simulink model "VariousSpeed2018_14dof_ypredictor_sc"  (R2017a)
settings: Solver=ode4  StartTime=0.0  StopTime=70  FixedStep=dt  RelTol=1e-3
values from neighbouring files (symbols this model uses):
  g_motor_eff = 1    [VESIM_init.m]
  gr_motor = 0    [VESIM_init.m]
undefined symbols (not defined in the file or in its folder): A_mc, brake_Pw, brake_V, C_q, diff_efficiency, diff_wRatio, dt, engine_inertia, error_lookuptable, F_cf, F_cs, fmin_mg, fmin_mg_na, J_cal, K_vb, Kp_rpm, mdot_fuel, model_lookuptable, no_cyl, P_0, P_gain, rpm0_c, rpm2rads, rpm_e, rpm_hi_idle, rpm_idle, rpm_max_c, rpm_rated, Standard_Devices, Ti_rpm, torque_engine, trq_scale, Tt_rpm, UDP_Protocol, vdes, Xobs, Yobs
libraries: simulink x10, vrlib x3, sldrtlib x3, SimulinkExecutionControl x1
(part 2 of 2)

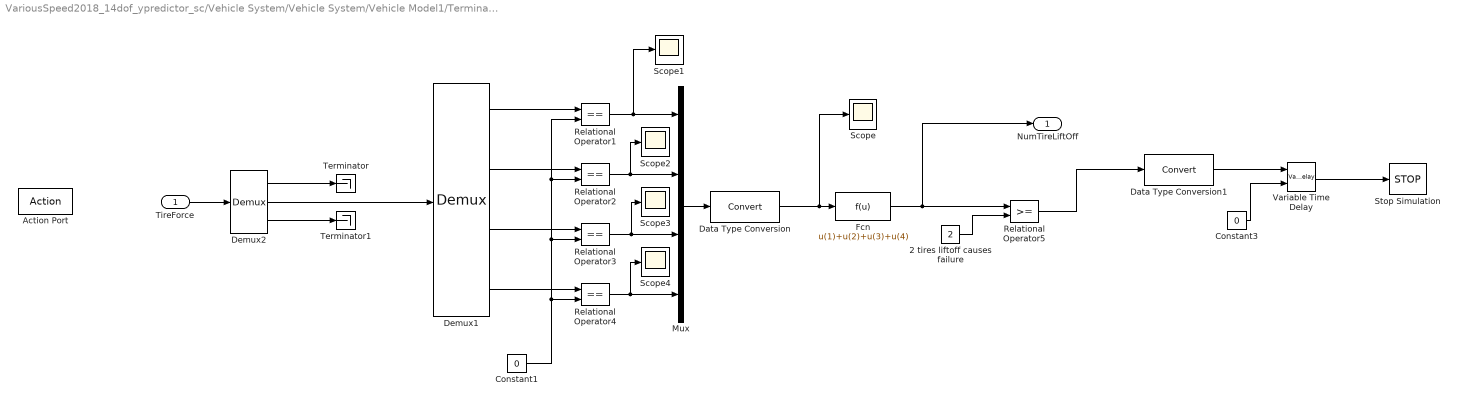
== system VariousSpeed2018_14dof_ypredictor_sc/Vehicle System/Vehicle System/Vehicle Model1/Terminate if vehicle tire lift-off ==
  TireForce : Inport
  Action Port : ActionPort
  2 tires liftoff causes failure : Constant  Value=2
  Constant1 : Constant  Value=0
  Constant3 : Constant  Value=0
  Data Type Conversion : DataTypeConversion
  Data Type Conversion1 : DataTypeConversion
  Demux1 : Demux
  Demux2 : Demux  Outputs=[8,4,17]
  Fcn : Fcn  Expr=u(1)+u(2)+u(3)+u(4)
  Mux : Mux
  Relational Operator{1..4} (4 alike) : RelationalOperator  Operator===  RndMeth=Nearest  InputSameDT=on
  Relational Operator5 : RelationalOperator  RndMeth=Nearest  InputSameDT=on
  Scope{,1..4} (5 alike) : Scope
  Stop Simulation : Stop
  Terminator : Terminator
  Terminator1 : Terminator
  Variable Time Delay : VariableTransportDelay  MaximumDelay=10  MaximumPoints=10000
  NumTireLiftOff : Outport  InitialOutput=0
  wires:
  Demux2/1 -> Terminator/1
  Demux2/3 -> Terminator1/1
  Demux2/2 -> Demux1/1
  TireForce/1 -> Demux2/1
  Demux1/1 -> Relational Operator1/1
  Demux1/2 -> Relational Operator2/1
  Demux1/3 -> Relational Operator3/1
  Demux1/4 -> Relational Operator4/1
  Relational Operator1/1 -> Scope1/1, Mux/1
  Relational Operator2/1 -> Scope2/1, Mux/2
  Relational Operator3/1 -> Scope3/1, Mux/3
  Relational Operator4/1 -> Scope4/1, Mux/4
  2 tires liftoff causes failure/1 -> Relational Operator5/2
  Mux/1 -> Data Type Conversion/1
  Data Type Conversion/1 -> Scope/1, Fcn/1
  Relational Operator5/1 -> Data Type Conversion1/1
  Constant1/1 -> Relational Operator2/2, Relational Operator1/2, Relational Operator3/2, Relational Operator4/2
  Fcn/1 -> NumTireLiftOff/1, Relational Operator5/1
  Variable Time Delay/1 -> Stop Simulation/1
  Constant3/1 -> Variable Time Delay/2
  Data Type Conversion1/1 -> Variable Time Delay/1

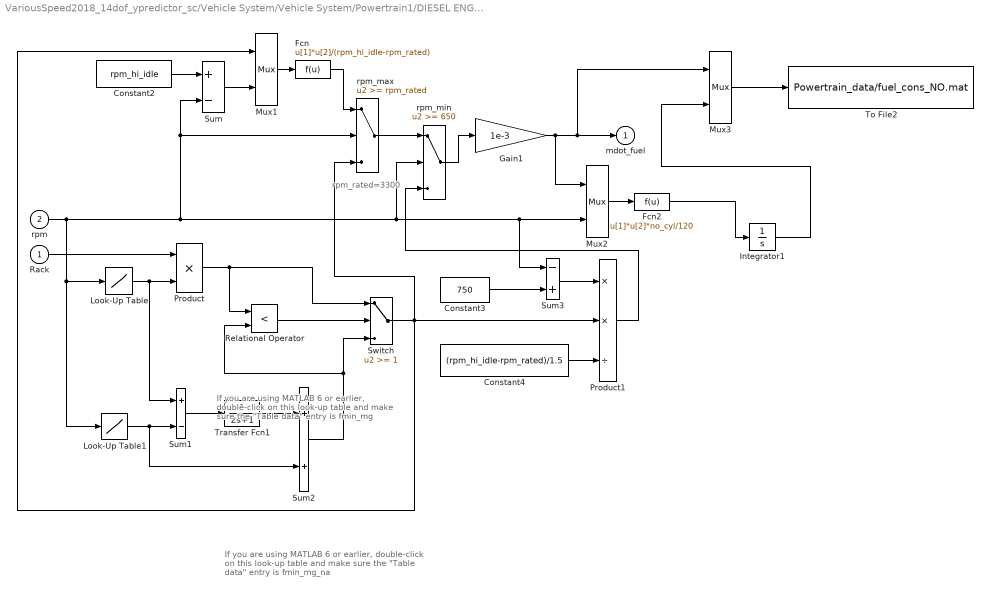
== system VariousSpeed2018_14dof_ypredictor_sc/Vehicle System/Vehicle System/Powertrain1/DIESEL ENGINE/Fuel controller// Governor ==
  note: If you are using MATLAB 6 or earlier,
      | double-click on this look-up table and
      | make sure the "Table data" entry is fmin_mg
  note: If you are using MATLAB 6 or earlier,
      | double-click on this look-up table and
      | make sure the "Table data" entry is fmin_mg_na
  note: rpm_rated=3300
  Rack : Inport
  rpm : Inport  Port=2
  Constant2 : Constant  Value=rpm_hi_idle
  Constant3 : Constant  Value=750
  Constant4 : Constant  Value=(rpm_hi_idle-rpm_rated)/1.5
  Fcn : Fcn  Expr=u[1]*u[2]/(rpm_hi_idle-rpm_rated)
  Fcn2 : Fcn  Expr=u[1]*u[2]*no_cyl/120
  Gain1 : Gain  Gain=1e-3  SaturateOnIntegerOverflow=on  OutDataTypeStr=Inherit: Same as input  ParamDataTypeStr=Inherit: Same as input
  Integrator1 : Integrator
  Look-Up Table : Lookup  InputValues=rpm_e  Table=fmin_mg  SaturateOnIntegerOverflow=on
  Look-Up Table1 : Lookup  InputValues=rpm_e  Table=fmin_mg_na  SaturateOnIntegerOverflow=on
  Mux1 : Mux  Inputs=2
  Mux2 : Mux  Inputs=2
  Mux3 : Mux  Inputs=2
  Product : Product  SaturateOnIntegerOverflow=on  InputSameDT=on  OutDataTypeStr=Inherit: Same as first input
  Product1 : Product  Inputs=**/  SaturateOnIntegerOverflow=on  InputSameDT=on  OutDataTypeStr=Inherit: Same as first input
  Relational Operator : RelationalOperator  Operator=<  RndMeth=Nearest  InputSameDT=on
  Sum : Sum  Inputs=+-  SaturateOnIntegerOverflow=on  InputSameDT=on  OutDataTypeStr=Inherit: Same as first input
  Sum1 : Sum  Inputs=+-  SaturateOnIntegerOverflow=on  InputSameDT=on  OutDataTypeStr=Inherit: Same as first input
  Sum2 : Sum  SaturateOnIntegerOverflow=on  InputSameDT=on  OutDataTypeStr=Inherit: Same as first input
  Sum3 : Sum  Inputs=-+  SaturateOnIntegerOverflow=on  InputSameDT=on  OutDataTypeStr=Inherit: Same as first input
  Switch : Switch  Threshold=1  SaturateOnIntegerOverflow=on  InputSameDT=on
  To File2 : ToFile  Filename=Powertrain_data/fuel_cons_NO.mat  MatrixName=fuel_cons
  Transfer Fcn1 : TransferFcn  Denominator=[2 1]
  rpm_max : Switch  Threshold=rpm_rated  SaturateOnIntegerOverflow=on  InputSameDT=on
  rpm_min : Switch  Threshold=650  SaturateOnIntegerOverflow=on  InputSameDT=on
  mdot_fuel : Outport  InitialOutput=0
  wires:
  Mux3/1 -> To File2/1
  Integrator1/1 -> Mux3/2
  Fcn2/1 -> Integrator1/1
  Switch/1 -> rpm_max/3, Product1/2, Mux1/1
  Product/1 -> Switch/1, Relational Operator/1
  Sum2/1 -> Relational Operator/2, Switch/3
  Relational Operator/1 -> Switch/2
  Look-Up Table1/1 -> Sum2/2, Sum1/2
  Transfer Fcn1/1 -> Sum2/1
  Look-Up Table/1 -> Product/2, Sum1/1
  Sum1/1 -> Transfer Fcn1/1
  Rack/1 -> Product/1
  rpm/1 -> rpm_max/2, Sum/2, Sum3/1, Mux2/2, rpm_min/2, Look-Up Table/1, Look-Up Table1/1
  Fcn/1 -> rpm_max/1
  rpm_max/1 -> rpm_min/1
  Product1/1 -> rpm_min/3
  Constant4/1 -> Product1/3
  Sum3/1 -> Product1/1
  Constant3/1 -> Sum3/2
  Constant2/1 -> Sum/1
  rpm_min/1 -> Gain1/1
  Mux2/1 -> Fcn2/1
  Gain1/1 -> Mux3/1, mdot_fuel/1, Mux2/1
  Sum/1 -> Mux1/2
  Mux1/1 -> Fcn/1

== system VariousSpeed2018_14dof_ypredictor_sc/Vehicle System/Vehicle System/Powertrain1/DIESEL ENGINE/Idle Controller ==
  note: 1/0.6464
  note: 2.7013
  note: 1/(3300-1000)
  note: 750 RPM
  note: anti-windup gain
  note: integral gain
  note: proportional gain
  engine speed : Inport
  driver command : Inport  Port=2
  Gain6 : Gain  Gain=Kp_rpm  SaturateOnIntegerOverflow=on  OutDataTypeStr=Inherit: Same as input  ParamDataTypeStr=Inherit: Same as input
  Gain7 : Gain  Gain=1/Ti_rpm  SaturateOnIntegerOverflow=on  OutDataTypeStr=Inherit: Same as input  ParamDataTypeStr=Inherit: Same as input
  Gain8 : Gain  Gain=1/(rpm_max_c-rpm0_c)  SaturateOnIntegerOverflow=on  OutDataTypeStr=Inherit: Same as input  ParamDataTypeStr=Inherit: Same as input
  Gain9 : Gain  Gain=1/Tt_rpm  SaturateOnIntegerOverflow=on  OutDataTypeStr=Inherit: Same as input  ParamDataTypeStr=Inherit: Same as input
  Idle speed : Constant  Value=rpm_idle
  Integrator2 : Integrator
  Saturation2 : Saturate  UpperLimit=1  LowerLimit=0.005
  Sum5 : Sum  Inputs=-+  SaturateOnIntegerOverflow=on  InputSameDT=on  OutDataTypeStr=Inherit: Same as first input
  Sum6 : Sum  SaturateOnIntegerOverflow=on  InputSameDT=on  OutDataTypeStr=Inherit: Same as first input
  Sum7 : Sum  Inputs=+-  SaturateOnIntegerOverflow=on  InputSameDT=on  OutDataTypeStr=Inherit: Same as first input
  Sum8 : Sum  SaturateOnIntegerOverflow=on  InputSameDT=on  OutDataTypeStr=Inherit: Same as first input
  Switch : Switch  Threshold=.11  SaturateOnIntegerOverflow=on  InputSameDT=on
  rack : Outport
  wires:
  Gain8/1 -> Gain6/1
  Sum7/1 -> Gain8/1
  engine speed/1 -> Sum7/2
  Idle speed/1 -> Sum7/1
  Saturation2/1 -> Sum5/2, rack/1
  driver command/1 -> Switch/2, Switch/1
  Switch/1 -> Sum5/1, Saturation2/1
  Sum6/1 -> Switch/3
  Gain9/1 -> Sum8/2
  Integrator2/1 -> Sum6/2
  Sum8/1 -> Integrator2/1
  Gain7/1 -> Sum8/1
  Sum5/1 -> Gain9/1
  Gain6/1 -> Gain7/1, Sum6/1

== system VariousSpeed2018_14dof_ypredictor_sc/Vehicle System/Vehicle System/Powertrain1/DRIVELINE/Drivetrain1 ==
  demand : Inport
  pump_f : Inport  Port=2
  shaft_f : Inport  Port=3
  Demux : Demux  Outputs=[1 1 1 1 1 1 1 1 1 1 1 1 1 ]
  Mux : Mux  Inputs=[1 1 1 ]
  S-Function : S-Function  FunctionName=Drivetrain  SFunctionDeploymentMode=off  EnableBusSupport=off
  gear_out : Outport
  gear_ratio_w : Outport  Port=2
  pump_e : Outport  Port=3
  shaft_e : Outport  Port=4
  stateDerTransC : Outport  Port=5
  stateDerTransI : Outport  Port=6
  stateTransC : Outport  Port=7
  stateTransI : Outport  Port=8
  trans_T_ratio_out : Outport  Port=9
  T_turbine_out : Outport  Port=10
  w_out_trans_out : Outport  Port=11
  w_ratio_disp : Outport  Port=12
  w_Turbine_out : Outport  Port=13
  wires:
  demand/1 -> Mux/1
  pump_f/1 -> Mux/2
  shaft_f/1 -> Mux/3
  Demux/1 -> gear_out/1
  Demux/2 -> gear_ratio_w/1
  Demux/3 -> pump_e/1
  Demux/4 -> shaft_e/1
  Demux/5 -> stateDerTransC/1
  Demux/6 -> stateDerTransI/1
  Demux/7 -> stateTransC/1
  Demux/8 -> stateTransI/1
  Demux/9 -> trans_T_ratio_out/1
  Demux/10 -> T_turbine_out/1
  Demux/11 -> w_out_trans_out/1
  Demux/12 -> w_ratio_disp/1
  Demux/13 -> w_Turbine_out/1
  Mux/1 -> S-Function/1
  S-Function/1 -> Demux/1

== system VariousSpeed2018_14dof_ypredictor_sc/Vehicle System/Vehicle System/Powertrain1/DRIVELINE/engine dynamics (flywheel inertia only) ==
  brake torque : Inport
  Load Torque : Inport  Port=2
  Engine polar moment of inertia1 : Constant  Value=engine_inertia
  Mux : Mux  Inputs=2
  Sum : Sum  Inputs=+-  SaturateOnIntegerOverflow=on  InputSameDT=on  OutDataTypeStr=Inherit: Same as first input
  calculate omega (replace current init val with value from input file) : Integrator  InitialCondition=0.01*2*pi/60
  div : Fcn  Expr=u[1]/u[2]
  rad/s : Outport  InitialOutput=0
  wires:
  Mux/1 -> div/1
  Sum/1 -> Mux/1
  Load Torque/1 -> Sum/2
  Engine polar moment of inertia1/1 -> Mux/2
  brake torque/1 -> Sum/1
  calculate omega (replace current init val with value from input file)/1 -> rad/s/1
  div/1 -> calculate omega (replace current init val with value from input file)/1

== matlab function VariousSpeed2018_14dof_ypredictor_sc/Autonomy/MATLAB Function4 ==
  data: u input; y output
function y = fcn(u)

y = u(u(104));

== matlab function VariousSpeed2018_14dof_ypredictor_sc/Autonomy/MATLAB Function ==
  data: u input; y output
function y = fcn(u)

y = u(min(u(104)+25,101));

== matlab function VariousSpeed2018_14dof_ypredictor_sc/Vehicle System/MATLAB Function ==
  data: u input; y output
function y = fcn(u)

y = 170*sin(0.005*u)+280*sin(0.001*u)+50*cos(0.02*u)-50;

== matlab function VariousSpeed2018_14dof_ypredictor_sc/Autonomy/MATLAB Function1 ==
  data: u input; y output
function y = fcn(u)
N = 51;
y = u(N+1);

== matlab function VariousSpeed2018_14dof_ypredictor_sc/Autonomy/MATLAB Function2 ==
  data: u input; y output
function y = fcn(u)

N = 51;
y = u(N+4);

== matlab function VariousSpeed2018_14dof_ypredictor_sc/Haptic Shared Control/Trigger1/MATLAB Function ==
  data: u input; vect output size=[1 10]; vect_old input; tr_vect_old input; threshold input; flag output; tr_vect output size=[1 20]; trigger output
function [vect, flag, tr_vect, trigger] = fcn(u, vect_old, tr_vect_old, threshold)
    vect = zeros(1,10); 
    vect(1,1) = u;
    vect(1,2:10) = vect_old(1:9);
    vect_ordered = sort(vect);
    
    if mean(vect_ordered(1:2)) > threshold
        flag = 1;
    else
        flag = 0;
    end
    
    tr_vect = zeros(1,20);
    tr_vect(1,1) = flag;
    tr_vect(1, 2:20) = tr_vect_old(1:19);
    if sum(tr_vect) == 20
        trigger = 1;
    else
        trigger = 0;
    end
end

== matlab function VariousSpeed2018_14dof_ypredictor_sc/Autonomy/Subsystem/Distance Indicator/Subsystem1/MATLAB Function ==
  data: Xv input; Xinit_final output; Yv input; Xinit input; alpha input; distance output
function [Xinit_final, distance] = DistanceIndicator(Xv, Yv, Xinit, alpha)

    threshold = 0.0005;
    Yinit = 170*sin(0.005*Xinit) + 280*sin(0.001*Xinit) + 50*cos(0.02*Xinit) - 50;
    Yd = 170*0.005*cos(0.005*Xinit) + 280*0.001*cos(0.001*Xinit) - 50*0.02*sin(0.02*Xinit);
    Ydd = -170*0.005*0.005*sin(0.005*Xinit) - 280*0.001*0.001*sin(0.001*Xinit) - 50*0.02*0.02*cos(0.02*Xinit);
    
    Proj = ((Xv - Xinit) + Yd * (Yv - Yinit))/sqrt(1 + Yd^2);
    Projd = (((-1 + Ydd * (Yv - Yinit) - (Yd)^2) * sqrt(1 + Yd^2)) - ((Xv - Xinit + Yd*(Yv - Yinit))) * 1/2 * (1+Yd^2)^(-1/2) * 2 * Yd * Ydd)/(1 + Yd^2);
    
    iter = 1;
    Move = 2 * Proj * Projd;
    
    while (abs(Move * alpha) >= threshold) && (iter <= 1000)
        Xinit = Xinit - alpha * Move;
        Yinit = 170*sin(0.005*Xinit) + 280*sin(0.001*Xinit) + 50*cos(0.02*Xinit) - 50;
        Yd = 170*0.005*cos(0.005*Xinit) + 280*0.001*cos(0.001*Xinit) - 50*0.02*sin(0.02*Xinit);
        Ydd = -170*0.005*0.005*sin(0.005*Xinit) - 280*0.001*0.001*sin(0.001*Xinit) - 50*0.02*0.02*cos(0.02*Xinit);
    
        Proj = ((Xv - Xinit) + Yd * (Yv - Yinit))/sqrt(1 + Yd^2);
        Projd = (((-1 + Ydd * (Yv - Yinit) - (Yd)^2) * sqrt(1 + Yd^2)) - ((Xv - Xinit + Yd*(Yv - Yinit))) * 1/2 * (1+Yd^2)^(-1/2) * 2 * Yd * Ydd)/(1 + Yd^2);
        Move = 2 * Proj * Projd;
        iter = iter + 1;
    end
    
    Xinit_final = Xinit;
    distance = sqrt((Xinit - Xv)^2 + (Yinit - Yv)^2);
end

== matlab function VariousSpeed2018_14dof_ypredictor_sc/Haptic Shared Control/Force Generator/Reference Governor/MATLAB Function ==
  data: ST_C input; ST_RG output; ST_L input
function ST_RG = fcn(ST_C, ST_L)
% ST_d = abs(ST_C - ST_L);
% if ST_d < 0.00075
%     ST_RG = ST_C;
% elseif ST_d < 0.00125
%     ST_RG = ST_L + 0.75*(ST_C - ST_L);
% elseif ST_d < 0.0016
%     ST_RG = ST_L + 0.5*(ST_C - ST_L);
% else
%     ST_RG = ST_L + 0.0016*(ST_C - ST_L)/ST_d;
ST_d = abs(ST_C - ST_L);
ST_diff = ST_C - ST_L;
    if ST_d < 0.0012
        ST_RG = ST_C;
    else
        add_diff = min(ST_d * 0.5, 0.0012) * ST_diff / ST_d;
        ST_RG = ST_L + add_diff;
    end

end

== matlab function VariousSpeed2018_14dof_ypredictor_sc/Vehicle System/Subsystem/MATLAB Function2 ==
  data: X0 input; ST_length input; X0predicted output; SP_length input; time_step input; idx input; dt input; st_old input; sp_old input
function X0predicted = fcn(X0, ST_length, SP_length, time_step, idx, dt, st_old, sp_old)
x0 = X0(1);
y0 = X0(2);
vy0 = X0(3);
dpsi = X0(4);
psi = X0(5);
if time_step == 0
    X0predicted = X0;
else
    if idx >= 1 
        st = ST_length(idx);
        vdes = SP_length(idx);
    else
        st = st_old;
        vdes = sp_old;
    end
    for i = 1:time_step
        four_dot = dotcalculator(st,vdes,x0,y0,vy0,dpsi,psi);
        if idx + i > 101
            st = ST_length(101);
            vdes = SP_length(101);
        else
            st = ST_length(idx+i);
            vdes = SP_length(idx+i);
        end
        x0 = x0 + dt * four_dot(1);
        y0 = y0 + dt * four_dot(2);
        vy0 = vy0 + dt * four_dot(3);
        dpsi = dpsi + dt * four_dot(4);
        psi = psi + dt * dpsi;
    end
    if idx + time_step > 101
        X0predicted = [x0; y0; vy0; dpsi; psi; ST_length(101); SP_length(101); 0];
    else
        a = idx+time_step;
        if a > 1
            X0predicted = [x0; y0; vy0; dpsi; psi; ST_length(a); SP_length(a); (SP_length(a) - SP_length(a-1))/dt];
        elseif a == 1
            X0predicted = [x0; y0; vy0; dpsi; psi; ST_length(a); SP_length(a); (SP_length(a) - sp_old)/dt];
        else
            X0predicted = [x0; y0; vy0; dpsi; psi; st_old; sp_old; (sp_old - vdes)/dt];
        end
    end
end
  


function fourdot = dotcalculator(st,vdes,x0,y0,vy0,dpsi,psi)
    % define model parameters
    m          = 2.6887e+03;
    Izz        = 4.1101e+03;
    la         = 1.5775;      % distance from CoG to front axle
    lb         = 1.7245;        % distance from CoG to rear axle
    FzF0       = 1.3680e+04;
    FzR0       = 1.2696e+04;
    dFzx_coeff = 705.;
    KZX        = 705.;
    KZYR       = 1040.;

    % defines polynominal for acceleration bounds
    AXC= [-0.000128015180401862,	0.00858618595422724,	-0.225657108071454,	3.08283259993589,	-0.000138537090018958,	0.00684702729623608,	-0.120391102052425,	-3.55886697370079];

    % vehicle Limits
    x_min    = 0.;
    x_max    = 400.;
    y_min    = 0.;
    y_max    = 400.;
    sa_min   = -30*pi/180;
    sa_max   = 30*pi/180;
    psi_min  = -2*pi;
    psi_max  = 2*pi;
    u_min    = 5.;   %5.
    u_max    = 29.;
    sr_min   = -5*pi/180;
    sr_max   = 5*pi/180;
    jx_min   = -5.;
    jx_max   = 5.;

    % tire parameters
    FZ0     = 35000.0;
    PCY1    = 1.5874;               %Shape factor Cfy for lateral forces
    PDY1    = 0.73957;              %Lateral friction Muy
    PDY2    = -0.075004;            %Variation of friction Muy with load
    PEY1    = 0.37562;              %Lateral curvature Efy at Fznom
    PEY2    = -0.069325;            %Variation of curvature Efy with load
    PEY3    = 0.29168;              %Zero order camber dependency of curvature Efy
    PKY1    = -10.289;              %Maximum value of stiffness Kfy/Fznom
    PKY2    = 3.3343;               %Load at which Kfy reaches maximum value
    PHY1    = 0.0056509;            %Horizontal shift Shy at Fznom
    PHY2    = -0.0020257;           %Variation of shift Shy with load
    PVY1    = 0.015216;             %Vertical shift in Svy/Fz at Fznom
    PVY2    = -0.010365;            %Variation of shift Svy/Fz with load
    PC1     = PCY1;
    PD1     = PDY1 - PDY2;
    PD2     = PDY2/FZ0;
    PE1     = PEY1 - PEY2;
    PE2     = PEY2/FZ0;
    PE3     = PEY3;
    PK1     = PKY1*FZ0;
    PK2     = 1/(PKY2*FZ0);
    PH1     = PHY1 - PHY2;
    PH2     = PHY2/FZ0;
    PV1     = PVY1 - PVY2;
    PV2     = PVY2/FZ0;

    Caf =  -8.4138e+04;	% cornering stiffness--front axle (N/rad)
    Car =  -7.8126e+04;	% cornering stiffness-- rear axle (N/rad)
    Fyf_min = -7500;
    Fyf_max = 7500;
    % constrained initial states
    x0_     = 0.;
    y0_     = 0.;
    psi0_   = 0.8464;
    v0_     = 0.;
    u0_     = 10.;
    sa0_    = 0.;
    sr0_    = 0.;
    ax0_    = 0.;
    jx0_    = 0.;
    r0_     = 0.;

    %%TODO: Move some of these parameters somewhere else
    % weights
    w_goal = 1.; % should be zero when vehicle is not within goal distance during prediction horizon
    w_psi  = 0.01;
    w_time = 0.05;
    w_haf  = 1.0e-5;
    w_Fz   = 0.1;  %0.5 in paper
    w_ce   = 1.;
    w_sa   = 0.1;
    w_sr   = 1.;
    w_jx   = 0.01;

    sm      = 5.; % (m) distance to make sure we don't hit obstacle
    Fz_min  = 1000.;
    Fz_off  = 100.;
    a_t     = Fz_min + 3*Fz_off;  % soft tire force constraint constants
    b_t     = Fz_off;
    EP      = 0.001;

    % other parameters
    L_Rd      = 5.;       % relaxation constant for LiDAR range (m)
    L_R       = 100.;     % LiDAR range (m)
    sigma     = 1.;       % 0.05 (m)small margin, if the vehicle is within this margin, then the target is considered to be reached

    
r=dpsi;    
v=vy0;    
ax=0;
ux=vdes;
sa=st;
FYF=( (PD2*(FzF0 - (ax - v*r)*dFzx_coeff)^2 + PD1*(FzF0 - (ax - v*r)*dFzx_coeff))*sin(PC1*atan((((PK1*sin(2*atan(PK2*(FzF0 - (ax - v*r)*dFzx_coeff))))/(((PD2*PC1*(FzF0 - (ax - v*r)*dFzx_coeff)^2 + PD1*PC1*(FzF0 - (ax - v*r)*dFzx_coeff)) + ((PD2*PC1*(FzF0 - (ax - v*r)*dFzx_coeff)^2 + PD1*PC1*(FzF0 - (ax - v*r)*dFzx_coeff)))/(((PD2*PC1*(FzF0 - (ax - v*r)*dFzx_coeff)^2 + PD1*PC1*(FzF0 - (ax - v*r)*dFzx_coeff))^2 + EP^2)^(0.5))*0.001)+EP))*((atan((v + la*r)/(ux+EP)) - sa) + PH2*(FzF0 - (ax - v*r)*dFzx_coeff) + PH1)) - ((PE2*(FzF0 - (ax - v*r)*dFzx_coeff) + PE1)*(1 - PE3)*(((atan((v + la*r)/(ux+EP)) - sa) + PH2*(FzF0 - (ax - v*r)*dFzx_coeff) + PH1))/((((atan((v + la*r)/(ux+EP)) - sa) + PH2*(FzF0 - (ax - v*r)*dFzx_coeff) + PH1)^2 + EP^2)^(0.5)))*((((PK1*sin(2*atan(PK2*(FzF0 - (ax - v*r)*dFzx_coeff))))/(((PD2*PC1*(FzF0 - (ax - v*r)*dFzx_coeff)^2 + PD1*PC1*(FzF0 - (ax - v*r)*dFzx_coeff)) + ((PD2*PC1*(FzF0 - (ax - v*r)*dFzx_coeff)^2 + PD1*PC1*(FzF0 - (ax - v*r)*dFzx_coeff)))/(((PD2*PC1*(FzF0 - (ax - v*r)*dFzx_coeff)^2 + PD1*PC1*(FzF0 - (ax - v*r)*dFzx_coeff))^2 + EP^2)^(0.5))*0.001)+EP))*((atan((v + la*r)/(ux+EP)) - sa) + PH2*(FzF0 - (ax - v*r)*dFzx_coeff) + PH1)) - atan((((PK1*sin(2*atan(PK2*(FzF0 - (ax - v*r)*dFzx_coeff))))/(((PD2*PC1*(FzF0 - (ax - v*r)*dFzx_coeff)^2 + PD1*PC1*(FzF0 - (ax - v*r)*dFzx_coeff)) + ((PD2*PC1*(FzF0 - (ax - v*r)*dFzx_coeff)^2 + PD1*PC1*(FzF0 - (ax - v*r)*dFzx_coeff)))/(((PD2*PC1*(FzF0 - (ax - v*r)*dFzx_coeff)^2 + PD1*PC1*(FzF0 - (ax - v*r)*dFzx_coeff))^2 + EP^2)^(0.5))*0.001)+EP))*((atan((v + la*r)/(ux+EP)) - sa) + PH2*(FzF0 - (ax - v*r)*dFzx_coeff) + PH1)))))) + (PV2*(FzF0 - (ax - v*r)*dFzx_coeff)^2 + PV1*(FzF0 - (ax - v*r)*dFzx_coeff)));
FYR=( (PD2*(FzR0 + (ax - v*r)*dFzx_coeff)^2 + PD1*(FzR0 + (ax - v*r)*dFzx_coeff))*sin(PC1*atan((((PK1*sin(2*atan(PK2*(FzR0 + (ax - v*r)*dFzx_coeff))))/(((PD2*PC1*(FzR0 + (ax - v*r)*dFzx_coeff)^2 + PD1*PC1*(FzR0 + (ax - v*r)*dFzx_coeff)) + ((PD2*PC1*(FzR0 + (ax - v*r)*dFzx_coeff)^2 + PD1*PC1*(FzR0 + (ax - v*r)*dFzx_coeff)))/(((PD2*PC1*(FzR0 + (ax - v*r)*dFzx_coeff)^2 + PD1*PC1*(FzR0 + (ax - v*r)*dFzx_coeff))^2+EP^2)^(0.5))*0.001)+EP))*((atan((v - lb*r)/(ux+EP))) + PH2*(FzR0 + (ax - v*r)*dFzx_coeff) + PH1)) - ((PE2*(FzR0 + (ax - v*r)*dFzx_coeff) + PE1)*(1 - PE3*(((atan((v - lb*r)/(ux+EP))) + PH2*(FzR0 + (ax - v*r)*dFzx_coeff) + PH1))/((((atan((v - lb*r)/(ux+EP))) + PH2*(FzR0 + (ax - v*r)*dFzx_coeff) + PH1)^2 + EP^2)^(0.5))))*((((PK1*sin(2*atan(PK2*(FzR0 + (ax - v*r)*dFzx_coeff))))/(((PD2*PC1*(FzR0 + (ax - v*r)*dFzx_coeff)^2 + PD1*PC1*(FzR0 + (ax - v*r)*dFzx_coeff)) + ((PD2*PC1*(FzR0 + (ax - v*r)*dFzx_coeff)^2 + PD1*PC1*(FzR0 + (ax - v*r)*dFzx_coeff)))/(((PD2*PC1*(FzR0 + (ax - v*r)*dFzx_coeff)^2 + PD1*PC1*(FzR0 + (ax - v*r)*dFzx_coeff))^2+EP^2)^(0.5))*0.001)+EP))*((atan((v - lb*r)/(ux+EP))) + PH2*(FzR0 + (ax - v*r)*dFzx_coeff) + PH1)) - atan((((PK1*sin(2*atan(PK2*(FzR0 + (ax - v*r)*dFzx_coeff))))/(((PD2*PC1*(FzR0 + (ax - v*r)*dFzx_coeff)^2 + PD1*PC1*(FzR0 + (ax - v*r)*dFzx_coeff)) + ((PD2*PC1*(FzR0 + (ax - v*r)*dFzx_coeff)^2 + PD1*PC1*(FzR0 + (ax - v*r)*dFzx_coeff)))/(((PD2*PC1*(FzR0 + (ax - v*r)*dFzx_coeff)^2 + PD1*PC1*(FzR0 + (ax - v*r)*dFzx_coeff))^2+EP^2)^(0.5))*0.001)+EP))*((atan((v - lb*r)/(ux+EP))) + PH2*(FzR0 + (ax - v*r)*dFzx_coeff) + PH1)))))) + (PV2*(FzR0 + (ax - v*r)*dFzx_coeff)^2 + PV1*(FzR0 + (ax - v*r)*dFzx_coeff)));
FZ_rl_con=(  0.5*(FzR0 + KZX*(ax - v*r)) - KZYR*((FYF + FYR)/m) - Fz_min);
FZ_rr_con=( 0.5*(FzR0 + KZX*(ax - v*r)) + KZYR*((FYF + FYR)/m) - Fz_min);



  xdot = ( vdes*cos(psi) - (v + la*r)*sin(psi));      % X position
  ydot= ( vdes*sin(psi) + (v + la*r)*cos(psi));        % Y position
  vydot = ((FYF + FYR)/m - r*ux);                    % Lateral Speed
  psiddot= ((la*FYF-lb*FYR)/Izz);                           % Yaw Rate
  fourdot=[xdot,ydot,vydot,psiddot];
end
end

== matlab function VariousSpeed2018_14dof_ypredictor_sc/Cognitive Workload Estimator/MATLAB Function ==
  data: u input; y output
function y = fcn(u)
if u<45
    y = 0;
elseif u>45 && u<75
    y = 0.5;
else
    y = 0;
end

== matlab function VariousSpeed2018_14dof_ypredictor_sc/Autonomy/MATLAB Function3 ==
  data: flagPrev output; Msg input; iter input; y output; sp output; yOld input; spOld input; t0 input; tStart output; uu output; AS_cnt_Old input; AS_cnt output; Setting input
% function [flagPrev,y, SolFeas,tStart] = fcn(Msg,iter,yOld,SolFeasPrev,t0)
function [flagPrev,y, sp, tStart, uu, AS_cnt] = fcn(Msg,iter,yOld,spOld,t0,AS_cnt_Old,Setting)
% u
% 1-31 st
% 32 comp_time
% 33 cmd_type
% 34 flag
% 35 iter_num
% 36 time_julia
% 37 data ready
% 38 st_hum
% 39 time_simulink

% Input length

tpred = 3;    % s
Npred = 31;     % #
t1 = linspace(0,tpred,Npred);
% Scale to ts = 0.01s
N = 301;
t2 = linspace(0,tpred,N);
uu = interp1(t1,Msg(1:Npred),t2)';
ss = interp1(t1,Msg(Npred+1:2*Npred),t2)';

% Execution window
Nexe = 101;
texe = (Nexe-1)*0.01;
u = [uu(1:Nexe);Msg(2*Npred+1:end)];
s = [ss(1:Nexe);Msg(2*Npred+1:end)];
pred_time = Msg(end-3)/100;

% Current time
t_sml = u(end);

% Initial outputs 
tStart = t0;
flagPrev = 0;
y = yOld;
sp = spOld;
AS_cnt = 0;

% Maximum Hold
MaxHold = 51;  % 0.5s to execute

% Initial case
if iter == 0
    y = u;
    y(1:Nexe) = u(end-1)*ones(Nexe,1);
    sp = s;
    sp(1:Nexe) = s(end-1)*ones(Nexe,1);
    y(Nexe+3) = 1;
    sp(Nexe+3) = 1;
    tStart = t0+0.01;
    return
end

switch Setting
    %% fix update version when optimal solution comes in, active safety
    case 1
        switch u(Nexe+2)
            % NOT OPTIMAL
            case {0,3}
                if yOld(Nexe+2) == 2
                    y = yOld;
                    sp = spOld;

                    y(Nexe+3) = y(Nexe+3)+1;
                    y(end) = u(end);
                    
                    sp(Nexe+3) = sp(Nexe+3)+1;
                    sp(end) = s(end);
                    
                    AS_cnt = AS_cnt_Old +1;
                    
                    if y(Nexe+3) > Nexe
                        y(1:Nexe) = -u(end-1)*ones(Nexe,1);
                        y(Nexe+3) = 1;
                        
                        sp(1:Nexe) = -s(end-1)*ones(Nexe,1);
                        sp(Nexe+3) = 1;
                        
                        AS_cnt = 0;
                        %y(Nexe+2) = 1;  % reset to human mode
                    end
                    
                else
                    y = u;
                    y(1:Nexe) = -u(end-1)*ones(Nexe,1);
                    y(Nexe+3) = 3;
                    
                    sp = s;
                    sp(1:Nexe) = -s(end-1)*ones(Nexe,1);
                    sp(Nexe+3) = 3;
                    
                    AS_cnt = 0;
                end
            % HUMAN FEASIBLE
            case 1
                if yOld(Nexe+2) == 2 && AS_cnt_Old < 10
                    y = yOld;
                    y(Nexe+3) = y(Nexe+3)+1;
                    
                    sp = spOld;
                    sp(Nexe+3) = sp(Nexe+3)+1;
                    
                    if y(Nexe+3) > Nexe
                        y(Nexe+3) = Nexe;
                        sp(Nexe+3) = Nexe;
                    end
                    y(end) = u(end);
                    sp(end) = s(end);
                    AS_cnt = AS_cnt_Old +1;
                else
                    y = u;
                    y(1:Nexe) = -u(end-1)*ones(Nexe,1);
                    
                    sp = s;
                    sp(1:Nexe) = -s(end-1)*ones(Nexe,1);
                    
                    AS_cnt = 0;
                 end
            % HUMAN INFEASIBLE, OPTIMAL
            case 2
                if yOld(Nexe+2) == 1 || yOld(Nexe+2) == 3
                    % Start first solution and execute it
                    AS_cnt = 1;
                    % Copy optimal solution from input
                    y = u;
                    sp = s;
                    t_julia = u(end-3);     
                    delay = t_sml - t_julia;
                    flagPrev = floor(delay/0.01)+2;
                    % Chop off signals
                    y(1:Nexe) = uu(flagPrev:(flagPrev+100));
                    sp(1:Nexe) = ss(flagPrev:(flagPrev+100));
                    % Shift the signals
                    y(1:Nexe) = y(1:Nexe) - (y(1)- (-u(end-1)) );
                    sp(1:Nexe) = sp(1:Nexe) - (sp(1)- (-s(end-1)) );
                %% Still in optimal solution
                else
                    % no new message
                    if u(end-2) == 0
                        y = yOld;
                        y(Nexe+3) = y(Nexe+3)+1;
                        
                        sp = spOld;
                        sp(Nexe+3) = sp(Nexe+3)+1;
                        
                        if y(Nexe+3) > Nexe
                            y(Nexe+3) = Nexe;
                            sp(Nexe+3) = Nexe;
                        end
                        y(end) = u(end);
                        sp(end) = s(end);
                        AS_cnt = AS_cnt_Old +1;
                        if AS_cnt_Old > MaxHold
                            AS_cnt = 1;
                        end
                    % new message, create a buffer
                    else
                        if AS_cnt_Old >= 10 || yOld(Nexe+4) == 1  % 1
                            AS_cnt = 1;
                            % Copy optimal solution from input
                            y = u;
                            sp = s;
                            t_julia = u(end-3);     
                            delay = t_sml - t_julia;
                            flagPrev = floor(delay/0.01)+2;
                            if flagPrev >= Nexe
                                flagPrev = Nexe;
                            end
                            % Chop off signals
                            y(1:Nexe) = uu(flagPrev:flagPrev+100);
                            % Shift the signals
                            y(1:Nexe) = y(1:Nexe) - (y(1)- yOld(yOld(Nexe+3)+1) );
                            
                            sp(1:Nexe) = ss(flagPrev:flagPrev+100);
                            % Shift the signals
                            sp(1:Nexe) = sp(1:Nexe) - (sp(1)- spOld(spOld(Nexe+3)+1) );
                        else
                            y = yOld;
                            y(Nexe+3) = y(Nexe+3)+1;
                            
                            sp = spOld;
                            sp(Nexe+3) = sp(Nexe+3)+1;
                            
                            if y(Nexe+3) > Nexe
                                y(Nexe+3) = Nexe;
                                sp(Nexe+3) = Nexe;
                            end
                            y(end) = u(end);
                            sp(end) = s(end);
                            AS_cnt = AS_cnt_Old +1;
                        end
                    end
                end
                
        end
      
    %% varying update version, haptic shared control    
    case {0,2,4}
%         if u(Nexe+2) == 3
%             if yOld(Nexe+2) == 2
%                 y = yOld;
%                 y(Nexe+3) = y(Nexe+3)+1;
%                 y(end) = u(end);
%                 
%                 sp = spOld;
%                 sp(Nexe+3) = sp(Nexe+3)+1;
%                 sp(end) = s(end);
% 
%                 if y(Nexe+3) > Nexe
%                     y(1:Nexe) = u(Nexe)*ones(Nexe,1);
%                     y(Nexe+3) = 1;
%                     
%                     sp(1:Nexe) = s(Nexe)*ones(Nexe,1);
%                     sp(Nexe+3) = 1;
%                     
%                     AS_cnt = 0;
%                    % y(Nexe+2) = 1;  % reset to human mode
%                 end        
%             else
%                 y = u;
%                 y(1:Nexe) = u(Nexe)*ones(Nexe,1);
%                 y(Nexe+3) = 1;
%                 
%                 sp = s;
%                 sp(1:Nexe) = s(Nexe)*ones(Nexe,1);
%                 sp(Nexe+3) = 1;
%             end
%             
%         else
            if u(end-5) > 0 
                y = u;  
                sp = s;  
                if u(Nexe+4) > 1
                    t_julia = u(end-4);     % time when vehicle is at, 7.21s, #38
                    delay = t_sml - t_julia;    % delay in vehicle state, 7.33-7.21
                    delay = delay - pred_time;
                    if delay < 0
                        delay = 0;
                    end
                    flagPrev = floor(delay/0.01)+1;
                    if flagPrev >=  Nexe
                        flagPrev = Nexe;
                    end
                else
                    flagPrev = 1;
                end
                % Chop off signals
                y(1:Nexe) = uu(flagPrev:(flagPrev+100));
                sp(1:Nexe) = ss(flagPrev:(flagPrev+100));
                % Shift the signals
%                 if yOld(Nexe+2) == 2
%                     y(1:Nexe) = y(1:Nexe) - (y(1)- yOld(yOld(Nexe+3)+1) );
%                 else
%                     y(1:Nexe) = y(1:Nexe) - (y(1)- (-u(end-1)) );
%                 end
                y(Nexe+3) = 1;
                sp(Nexe+3) = 1;
                
                % fight exists and automation complies
%                 if abs(y(1)- (-u(end-1)) ) >= 0.025   % 0.03
%                     y(1:Nexe) = -u(end-1)*ones(Nexe,1);
% %                    y(Nexe+2) = 1;
%                 end

            else
                % Continue previous solution
%                 if yOld(Nexe+2) == 2
                    y = yOld;
                    sp = spOld;
                    % Increase flag
                    y(Nexe+3) = y(Nexe+3)+1;
                    
                    sp(Nexe+3) = sp(Nexe+3)+1;
                    
                    if y(Nexe+3) > Nexe
                        y(Nexe+3) = Nexe;
                        y(end-1) = u(end-1);
                        
                        sp(Nexe+3) = Nexe;
                        sp(end-1) = s(end-1);
                    end
                    y(end) = u(end);
                    sp(end) = s(end);
                % Use human command
%                 else
%                     y = yOld;
%                     y(1:Nexe) = u(end-1)*ones(Nexe,1);
%                     y(Nexe+3) = y(Nexe+3)+1;
%                     if y(Nexe+3) > Nexe
%                         y(Nexe+3) = Nexe;
%                         y(end-1) = u(end-1);
%                     end
%                     y(end) = u(end);
%                 end
            end
%         end
    
    %% teleoperation
    case 3
        y = u;
        y(1:Nexe) = -u(end-1)*ones(Nexe,1);
        y(Nexe+3) = 1;
        
        sp = s;
        sp(1:Nexe) = -s(end-1)*ones(Nexe,1);
        sp(Nexe+3) = 1;
              
        
        
        
    %% fixed update version  
    case 5
        % Update every texe
        if mod(t_sml-tStart+0.01,texe) >= texe || mod(t_sml-tStart+0.01,texe) < 0.01  
            % Find the latest feasible solution if the current one is
            % infeasible ,need ++++ 
%             if u(Nexe+2) == 3
%                 u = SolFeasPrev;
%             end
            t_julia = u(end-3);     % time when vehicle is at, 7.32s
            y = u; % new input, #39
            sp = s;
            
            if u(Nexe+4) > 1   % need prediction
                delay = t_sml - t_julia;    % delay in vehicle state, 7.69-7.32
                flagPrev = floor(delay/0.01)+1;    
            else
                flagPrev = 1;
            end
            if flagPrev >=  Nexe
                flagPrev = Nexe;
            end

            % prediction
            y(1:Nexe) = uu(flagPrev:(flagPrev+100));
            sp(1:Nexe) = ss(flagPrev:(flagPrev+100));
            disp('Predict')
        else
            y = yOld;
            sp = spOld;
            % Increase flag
            y(Nexe+3) = y(Nexe+3)+1;
            sp(Nexe+3) = sp(Nexe+3)+1;
            if y(Nexe+3) > Nexe
                y(Nexe+3) = Nexe;
                y(end-1) = u(end-1);
                sp(Nexe+3) = Nexe;
                sp(end-1) = s(end-1);
            end
            y(end) = u(end);
            sp(end) = s(end);
        end
        
end
                    
end

== matlab function VariousSpeed2018_14dof_ypredictor_sc/Autonomy/Subsystem/Subsystem/MATLAB Function ==
  data: XG input; Xobs_pass output; Yobs_pass output; YG input; PHIG input; Xobs input; Yobs input; vdes input
function [Xobs_pass,Yobs_pass] = fcn(XG,YG,PHIG,Xobs,Yobs,vdes)
    Xobs_seen = Xobs(1:8);
    Yobs_seen = Yobs(1:8);
    N = length(Xobs_seen);
    Xveh = XG*ones(N,1);
    Yveh = YG*ones(N,1);
    ObsR = 1*ones(N,1);
    sm = 2;
    Dist = sqrt( (Xveh-Xobs_seen).^2+(Yveh-Yobs_seen).^2 );
    Dir = atan2(Yobs_seen-Yveh, Xobs_seen-Xveh );
    % find front and out of safe margin, else 0
    ActiveAll = double(abs(Dir-PHIG)<=pi/2 & Dist>=ObsR+sm & Dist <=10*vdes );    
    
    Dist = Dist.* ActiveAll;
    for i = 1:length(Dist)
        if Dist(i) == 0
            Dist(i) = 2000;
        end
    end
    [Distsort,sortIdx] = sort(Dist);
    InvalidAll = double(Distsort == 2000);
    
    % Obstacles in the front 
    Xobs_inview = Xobs(sortIdx)+InvalidAll*900;
    Yobs_inview = Yobs(sortIdx)+InvalidAll*900;
    
    Xobs_pass = Xobs_inview(1:3);
    Yobs_pass = Yobs_inview(1:3);

== matlab function VariousSpeed2018_14dof_ypredictor_sc/Autonomy/MATLAB Function5 ==
  data: u input; y output
function y = fcn(u)

y = u(min(u(104)+25,101));

== matlab function VariousSpeed2018_14dof_ypredictor_sc/Haptic Shared Control/Subsystem2/MATLAB Function ==
  data: theta input; thetad input; athetadd input; F_p output
function F_p = force_prediction(theta, thetad, athetadd)
% bi-section
init_1 = -0.4228;
init_2 = 0.4386;
sol_tol = 0.0001;

while abs(init_1 - init_2) > sol_tol
    med = (init_1 + init_2)/2;
    if abs(generate_solution(init_1, theta, athetadd, thetad)) < 0.0001
        init_2 = init_1;
    elseif abs(generate_solution(init_2, theta, athetadd, thetad)) < 0.0001
        init_1 = init_2; 
    elseif generate_solution(init_1, theta, athetadd, thetad)*generate_solution(med, theta, athetadd, thetad) <= 0
        init_2 = med;
    else
        init_1 = med;
    end    
end
F_p = (init_1 + init_2)/2;

    function sol = generate_solution(F, theta, athetadd, thetad)
        sol = F + athetadd - generate_b(F, theta)*thetad;
    end

    function b = generate_b(F, theta)
        eval_F = [-0.70 ,-0.60, -0.57, -0.55, -0.52, -0.50, -0.47, -0.45, -0.42, -0.40, -0.39, -0.38, -0.37, -0.36, -0.35, -0.34, -0.33, -0.32, -0.31, -0.30, -0.29, -0.28, -0.27, -0.26, -0.25, -0.24, -0.23, -0.22, -0.21, -0.20, -0.19, 0.17, 0.18, 0.19, 0.20, 0.21, 0.22, 0.23, 0.24, 0.25, 0.26, 0.27, 0.28, 0.29, 0.30, 0.31, 0.32, 0.33, 0.34, 0.35, 0.36, 0.37, 0.38, 0.39, 0.40, 0.42, 0.45, 0.47, 0.50, 0.52, 0.55, 0.57, 0.60];
        eval_F = eval_F + ((eval_F<0).*+0.1772 + (eval_F>0).*-0.1614);
        eval_theta = [-0.16, -0.15, -0.13, -0.11, -0.09, -0.07, -0.05, -0.03, -0.01, 0, 0.01, 0.03, 0.05, 0.07, 0.09, 0.11, 0.13, 0.15, 0.16];
        b_ref = [...
             7.0467, 5.2850, 3.5233, 2.7277, 2.4252, 2.2078, 1.9896, 2.1133, 1.4272, 1.4464, 1.8675, 1.6168, 1.9454, 2.1594, 2.3480, 2.7159, 3.5293, 4.9741, 10.5700;...%-0.70
             7.0467, 5.2850, 3.5233, 2.7277, 2.4252, 2.2078, 1.9896, 2.1133, 1.4272, 1.4464, 1.8675, 1.6168, 1.9454, 2.1594, 2.3480, 2.7159, 3.5293, 4.9741, 10.5700;...%-0.60
             6.0431, 4.9100, 3.2733, 2.8057, 2.1523, 2.1348, 1.7575, 1.7497, 1.6411, 1.6134, 1.6238, 1.7115, 1.8705, 1.9838, 2.3312, 2.6187, 3.0659, 5.2373, 10.2933;...%-0.57
             6.2133, 5.3257, 3.2256, 2.5710, 2.2250, 2.0372, 1.8230, 1.6423, 1.5415, 1.5213, 1.5313, 1.6387, 1.7966, 1.7923, 2.2323, 2.5710, 3.1954, 4.9707, 7.4560;...%-0.55
             6.8560, 3.9111, 2.9809, 2.3641, 2.1235, 1.9151, 1.5653, 1.5653, 1.5325, 1.4172, 1.4612, 1.5582, 1.6887, 1.7055, 2.0239, 2.4486, 3.1164, 4.5707, 8.5700;...%-0.52
             6.4560, 4.3040, 2.9345, 2.3057, 2.0430, 1.8446, 1.6554, 1.5102, 1.3914, 1.3884, 1.4220, 1.4541, 1.6221, 1.7834, 2.0826, 2.3911, 2.8070, 4.4524, 7.4492;...%-0.50
             4.8800, 3.9927, 2.6618, 2.0914, 1.9013, 1.5853, 1.5411, 1.4283, 1.3225, 1.3035, 1.2944, 1.3910, 1.5250, 1.6358, 1.9520, 2.0914, 2.4618, 4.1829, 7.7600;...%-0.47
             6.8200, 3.4100, 2.6231, 2.0985, 1.6934, 1.6884, 1.4826, 1.3438, 1.2595, 1.2495, 1.2485, 1.3147, 1.4588, 1.5333, 1.8187, 2.0224, 2.7280, 3.7628, 6.8200;...%-0.45
             4.8560, 3.4686, 2.3124, 1.8677, 1.6687, 1.3679, 1.3640, 1.2451, 1.1444, 1.1283, 1.1453, 1.1961, 1.3196, 1.4715, 1.6716, 1.8677, 2.4280, 3.4686, 5.3956;...%-0.42
             4.4560, 3.1829, 2.2280, 1.7138, 1.5690, 1.3288, 1.2731, 1.1726, 1.0226, 1.0665, 1.0900, 1.1367, 1.2117, 1.4101, 1.5201, 1.8567, 2.2280, 3.7133, 4.0509;...%-0.40
             4.5106, 3.5467, 2.1280, 1.6369, 1.4986, 1.3641, 1.2160, 1.1141, 0.9372, 1.0109, 0.9776, 1.0885, 1.1955, 1.2251, 1.4812, 1.7733, 2.1280, 3.0400, 5.3200;...%-0.39
             4.3800, 3.3800, 1.9314, 1.8436, 1.5364, 1.4182, 1.2675, 1.1523, 1.0562, 1.0496, 1.0607, 1.1122, 1.2291, 1.3703, 1.5600, 1.6900, 2.0280, 3.3800, 6.7600;...%-0.38
             9.6400, 3.2133, 1.9280, 1.7527, 1.5424, 1.3251, 1.2280, 1.1209, 1.0377, 1.0145, 1.0205, 1.0955, 1.1803, 1.2205, 1.5224, 1.7527, 2.1100, 3.0560, 6.8200;...%-0.37
             9.1400, 3.0467, 2.2850, 1.6618, 1.4862, 1.3642, 1.2106, 1.1012, 1.0184, 0.9779, 1.0270, 1.0381, 1.1794, 1.2151, 1.4822, 1.6618, 2.2850, 3.0060, 5.5700;...%-0.36
             4.3200, 3.4560, 2.1600, 1.7280, 1.5429, 1.4400, 1.2706, 1.1597, 1.0654, 1.0378, 1.0673, 1.0148, 1.2432, 1.3606, 1.6000, 1.7280, 2.1600, 3.2560, 5.7600;...%-0.35
             8.1400, 3.2560, 2.0350, 1.6280, 1.5654, 1.4157, 1.2921, 1.1587, 1.0682, 1.0365, 1.0696, 1.0926, 1.2241, 1.3681, 1.5505, 1.6089, 2.3257, 3.2560, 5.4267;...%-0.34
             5.0933, 3.0560, 2.1829, 1.6978, 1.5434, 1.4018, 1.2628, 1.1319, 1.0596, 1.0349, 1.0480, 1.0685, 1.2031, 1.3287, 1.5280, 1.6978, 2.1829, 3.0560, 5.0933;...%-0.33
             4.7600, 2.8560, 2.0400, 1.7850, 1.4875, 1.2865, 1.2102, 1.0901, 1.0340, 0.9882, 1.0099, 1.0200, 1.1802, 1.3346, 1.4875, 1.7850, 2.0400, 3.1733, 4.7600;...%-0.32
             5.3120, 2.9511, 2.4560, 1.7707, 1.5810, 1.4593, 1.3020, 1.2893, 0.9124, 1.0703, 1.2051, 1.1021, 1.1964, 1.3621, 1.7826, 1.8971, 2.0145, 3.0271, 6.6400;...%-0.31
             6.1400, 2.7289, 2.2327, 1.7543, 1.7175, 1.2792, 1.2926, 1.1423, 1.0285, 1.0422, 1.1825, 1.0586, 1.1922, 1.3569, 1.5336, 1.7543, 2.0467, 3.0086, 4.9120;...%-0.30
             3.7600, 3.0229, 2.2260, 1.7500, 1.5040, 1.3756, 1.2129, 1.2261, 0.9956, 0.9907, 1.0236, 0.9616, 1.1510, 1.2966, 1.3429, 1.7905, 2.0560, 3.0878, 5.6400;...%-0.29
             6.2800, 3.2267, 2.0560, 1.7133, 1.6062, 1.4899, 1.2850, 1.1953, 1.0576, 1.0388, 1.0708, 1.0821, 1.2094, 1.3892, 1.5118, 1.8691, 2.2844, 3.2267, 5.1400;...%-0.28
             4.6400, 3.2400, 2.2622, 1.7467, 1.6000, 1.4730, 1.3449, 1.2052, 1.1127, 1.0941, 1.1317, 1.1317, 1.2541, 1.4061, 1.6000, 1.8560, 2.3200, 3.0933, 4.6400;...%-0.27
             4.1400, 2.7600, 2.0700, 1.7700, 1.5923, 1.4526, 1.2738, 1.1500, 1.1753, 1.0336, 1.1355, 1.0753, 1.2795, 1.2938, 1.5623, 1.7560, 2.1700, 2.8600, 5.1400;...%-0.26
             3.6400, 2.9120, 1.8200, 1.4560, 1.3736, 1.1648, 1.2661, 0.9973, 0.9455, 0.8999, 0.9122, 0.9455, 1.0628, 1.1742, 1.3736, 1.8200, 2.0800, 2.9120, 3.6400;...%-0.25
             3.1400, 3.1400, 2.0933, 1.5700, 1.4273, 1.2816, 1.2077, 1.0555, 0.9508, 0.9191, 0.9458, 0.9662, 1.0467, 1.1849, 1.3802, 1.5700, 2.0933, 2.0933, 6.2800;...%-0.24
             5.2800, 2.6400, 1.7600, 1.3200, 1.3538, 1.2878, 1.2000, 1.0154, 0.9412, 0.9085, 1.0312, 0.9263, 1.0154, 1.1234, 1.2878, 1.7600, 1.7600, 2.6400, 4.6400;...%-0.23
             6.4800, 2.1400, 1.4267, 1.4267, 1.2970, 1.0700, 1.0974, 0.9304, 0.7329, 0.8013, 0.8231, 0.7782, 0.9106, 1.0439, 1.1889, 1.4267, 1.4267, 2.1400, 6.4800;...%-0.22
             4.6800, 2.1867, 1.6400, 1.3120, 1.0933, 1.0092, 1.0933, 0.8000, 0.7736, 0.6961, 0.7472, 0.6979, 0.7904, 0.8865, 1.0754, 1.0933, 1.3120, 2.1867, 4.6800;...%-0.21
             4.5600, 2.2800, 1.3680, 1.1400, 1.0688, 1.0364, 1.0133, 0.7475, 0.7475, 0.6598, 0.7331, 0.6706, 0.7125, 0.8769, 1.0364, 1.1400, 1.1400, 2.2800, 4.5600;...%-0.20
             2.5600, 1.9200, 1.2800, 0.8533, 0.8000, 0.7529, 0.8000, 0.5818, 0.5447, 0.4288, 0.5110, 0.4491, 0.5020, 0.6095, 0.7420, 0.8533, 1.2800, 1.2800, 2.8400;...%-0.19

             0.9801, 0.8696, 0.6484, 0.4987, 0.4596, 0.4598, 0.4465, 0.3984, 0.3501, 0.3501, 0.3501, 0.3984, 0.4465, 0.4598, 0.4596, 0.4987, 0.6484, 0.8696, 0.9801;...
             1.9013, 1.6674, 1.1997, 0.8794, 0.7967, 0.8043, 0.7629, 0.6781, 0.5997, 0.5997, 0.5997, 0.6781, 0.7629, 0.8043, 0.7967, 0.8794, 1.1997, 1.6674, 1.9013;...
             2.0337, 1.8431, 1.4617, 1.1568, 1.0182, 0.9695, 0.9481, 0.8350, 0.7578, 0.7578, 0.7578, 0.8350, 0.9481, 0.9695, 1.0182, 1.1568, 1.4617, 1.8431, 2.0337;...
             2.7919, 2.4495, 1.7646, 1.3272, 1.1971, 1.1264, 1.0362, 0.9966, 0.9079, 0.9079, 0.9079, 0.9966, 1.0362, 1.1264, 1.1971, 1.3272, 1.7646, 2.4495, 2.7919;...
             2.6983, 2.4057, 1.8203, 1.3931, 1.2182, 1.1377, 1.0665, 0.9688, 0.8972, 0.8972, 0.8972, 0.9688, 1.0665, 1.1377, 1.2182, 1.3931, 1.8203, 2.4057, 2.6983;...
             2.8268, 2.4864, 1.8054, 1.4162, 1.3061, 1.1838, 1.0953, 0.9767, 0.9612, 0.9612, 0.9612, 0.9767, 1.0953, 1.1838, 1.3061, 1.4162, 1.8054, 2.4864, 2.8268;...
             2.8584, 2.5726, 2.0009, 1.5802, 1.3832, 1.2587, 1.1828, 1.0554, 1.0217, 1.0217, 1.0217, 1.0554, 1.1828, 1.2587, 1.3832, 1.5802, 2.0009, 2.5726, 2.8584;...
             3.1268, 2.7998, 2.1458, 1.6240, 1.3987, 1.3380, 1.2281, 1.1229, 1.1032, 1.1032, 1.1032, 1.1229, 1.2281, 1.3380, 1.3987, 1.6240, 2.1458, 2.7998, 3.1268;...
             3.0939, 2.8127, 2.2502, 1.7899, 1.5427, 1.4063, 1.3126, 1.1836, 1.1684, 1.1684, 1.1684, 1.1836, 1.3126, 1.4063, 1.5427, 1.7899, 2.2502, 2.8127, 3.0939;...
             3.4414, 3.0741, 2.3394, 1.7942, 1.5645, 1.4607, 1.3507, 1.2325, 1.1952, 1.1952, 1.1952, 1.2325, 1.3507, 1.4607, 1.5645, 1.7942, 2.3394, 3.0741, 3.4414;...
             3.2580, 2.9865, 2.4435, 1.8965, 1.5765, 1.4877, 1.3834, 1.2852, 1.2567, 1.2567, 1.2567, 1.2852, 1.3834, 1.4877, 1.5765, 1.8965, 2.4435, 2.9865, 3.2580;...
             2.9194, 2.6457, 2.0983, 1.6849, 1.4794, 1.3477, 1.2419, 1.1404, 1.1459, 1.1459, 1.1459, 1.1404, 1.2419, 1.3477, 1.4794, 1.6849, 2.0983, 2.6457, 2.9194;...
             3.2287, 2.9003, 2.2437, 1.7614, 1.5376, 1.3978, 1.2796, 1.1534, 1.2036, 1.2036, 1.2036, 1.1534, 1.2796, 1.3978, 1.5376, 1.7614, 2.2437, 2.9003, 3.2287;...
             3.3586, 3.0139, 2.3247, 1.8108, 1.5683, 1.4215, 1.3075, 1.2158, 1.2260, 1.2260, 1.2260, 1.2158, 1.3075, 1.4215, 1.5683, 1.8108, 2.3247, 3.0139, 3.3586;...
             2.9721, 2.7244, 2.2290, 1.7890, 1.5295, 1.3953, 1.2866, 1.2383, 1.2425, 1.2425, 1.2425, 1.2383, 1.2866, 1.3953, 1.5295, 1.7890, 2.2290, 2.7244, 2.9721;...
             3.4207, 3.0320, 2.2546, 1.7260, 1.4961, 1.3162, 1.2439, 1.1662, 1.2200, 1.2200, 1.2200, 1.1662, 1.2439, 1.3162, 1.4961, 1.7260, 2.2546, 3.0320, 3.4207;...
             3.2041, 2.8989, 2.2887, 1.7759, 1.5120, 1.3992, 1.2677, 1.1832, 1.2836, 1.2836, 1.2836, 1.1832, 1.2677, 1.3992, 1.5120, 1.7759, 2.2887, 2.8989, 3.2041;...
             3.2228, 2.8871, 2.2157, 1.7518, 1.5386, 1.3686, 1.2446, 1.1711, 1.2725, 1.2725, 1.2725, 1.1711, 1.2446, 1.3686, 1.5386, 1.7518, 2.2157, 2.8871, 3.2228;...
             3.0441, 2.7794, 2.2500, 1.8127, 1.5556, 1.3868, 1.2700, 1.1899, 1.2573, 1.2573, 1.2573, 1.1899, 1.2700, 1.3868, 1.5556, 1.8127, 2.2500, 2.7794, 3.0441;...
             3.0736, 2.7780, 2.1869, 1.7530, 1.5345, 1.3744, 1.2731, 1.1648, 1.1540, 1.1540, 1.1540, 1.1648, 1.2731, 1.3744, 1.5345, 1.7530, 2.1869, 2.7780, 3.0736;...
             3.0118, 2.7329, 2.1753, 1.7180, 1.4749, 1.3458, 1.2199, 1.1557, 1.2307, 1.2307, 1.2307, 1.1557, 1.2199, 1.3458, 1.4749, 1.7180, 2.1753, 2.7329, 3.0118;...
             3.1563, 2.8641, 2.2795, 1.8063, 1.5536, 1.4103, 1.2821, 1.2035, 1.3169, 1.3169, 1.3169, 1.2035, 1.2821, 1.4103, 1.5536, 1.8063, 2.2795, 2.8641, 3.1563;...
             3.4738, 3.0816, 2.2972, 1.8250, 1.6502, 1.4607, 1.3939, 1.2630, 1.3607, 1.3607, 1.3607, 1.2630, 1.3939, 1.4607, 1.6502, 1.8250, 2.2972, 3.0816, 3.4738;...
             3.4012, 3.0696, 2.4064, 1.8896, 1.6348, 1.4959, 1.3557, 1.3074, 1.4815, 1.4815, 1.4815, 1.3074, 1.3557, 1.4959, 1.6348, 1.8896, 2.4064, 3.0696, 3.4012;...
             3.3487, 3.0668, 2.5030, 2.0545, 1.7957, 1.6112, 1.4693, 1.3792, 1.5550, 1.5550, 1.5550, 1.3792, 1.4693, 1.6112, 1.7957, 2.0545, 2.5030, 3.0668, 3.3487;...
             4.0084, 3.6076, 2.8058, 2.2011, 1.8973, 1.6976, 1.5901, 1.4724, 1.6255, 1.6255, 1.6255, 1.4724, 1.5901, 1.6976, 1.8973, 2.2011, 2.8058, 3.6076, 4.0084;...
             4.1272, 3.7126, 2.8834, 2.2985, 2.0152, 1.7890, 1.5948, 1.5240, 1.6681, 1.6681, 1.6681, 1.5240, 1.5948, 1.7890, 2.0152, 2.2985, 2.8834, 3.7126, 4.1272;...
             4.5238, 4.0440, 3.0844, 2.4310, 2.1407, 1.9076, 1.6846, 1.6397, 1.7968, 1.7968, 1.7968, 1.6397, 1.6846, 1.9076, 2.1407, 2.4310, 3.0844, 4.0440, 4.5238;...
             4.7290, 4.2519, 3.2976, 2.5859, 2.2411, 2.0203, 1.8677, 1.7366, 1.8974, 1.8974, 1.8974, 1.7366, 1.8677, 2.0203, 2.2411, 2.5859, 3.2976, 4.2519, 4.7290;...
             5.3025, 4.6965, 3.4845, 2.6168, 2.2838, 2.1410, 2.0187, 1.8287, 1.9626, 1.9626, 1.9626, 1.8287, 2.0187, 2.1410, 2.2838, 2.6168, 3.4845, 4.6965, 5.3025;...
             5.2534, 4.6697, 3.5023, 2.6938, 2.3666, 2.1619, 1.9228, 1.8658, 1.9739, 1.9739, 1.9739, 1.8658, 1.9228, 2.1619, 2.3666, 2.6938, 3.5023, 4.6697, 5.2534;...
             5.6391, 5.0126, 3.7595, 2.8304, 2.4448, 2.2784, 2.1395, 1.9668, 2.0836, 2.0836, 2.0836, 1.9668, 2.1395, 2.2784, 2.4448, 2.8304, 3.7595, 5.0126, 5.6391;
            ];
        idx = min(find(F<=eval_F));
        jdx = min(find(theta<=eval_theta));
        if F == eval_F(idx)
            b_ref_u = b_ref(idx, :);
        else
            b_ref_u = b_ref(idx-1,:) + (b_ref(idx,:)-b_ref(idx-1,:))/(eval_F(idx)-eval_F(idx-1))*(F-eval_F(idx-1));
        end
        if theta == eval_theta(jdx)
            b = b_ref_u(jdx);
        else
            b = b_ref_u(jdx-1) + (b_ref_u(jdx)-b_ref_u(jdx-1))/(eval_theta(jdx)-eval_theta(jdx-1))*(theta-eval_theta(jdx-1));
        end
    end

end

== matlab function VariousSpeed2018_14dof_ypredictor_sc/Haptic Shared Control/Subsystem2/MATLAB Function1 ==
  data: F input; b input; J_cal input; theta_p output; theta input; thetad input; dt input
function theta_p = theta_prediction(F, b, J_cal, theta, thetad, dt)
    if b == 0 
        b = 10;
    end
    c_2 = (thetad-(F/b))/(-b/J_cal);
    c_1 = theta - c_2;
    theta_p = c_1 + c_2 * exp((-b/J_cal)*dt) + F/b*dt;
end
